simulink model "pressingswitch_fan"  (R2021a)
settings: Solver=FixedStepAuto  StartTime=0.0  StopTime=inf  FixedStep=0.01  RelTol=1e-3
libraries: simulink x1
settings Model: Creator=surya  LastModifiedBy=surya

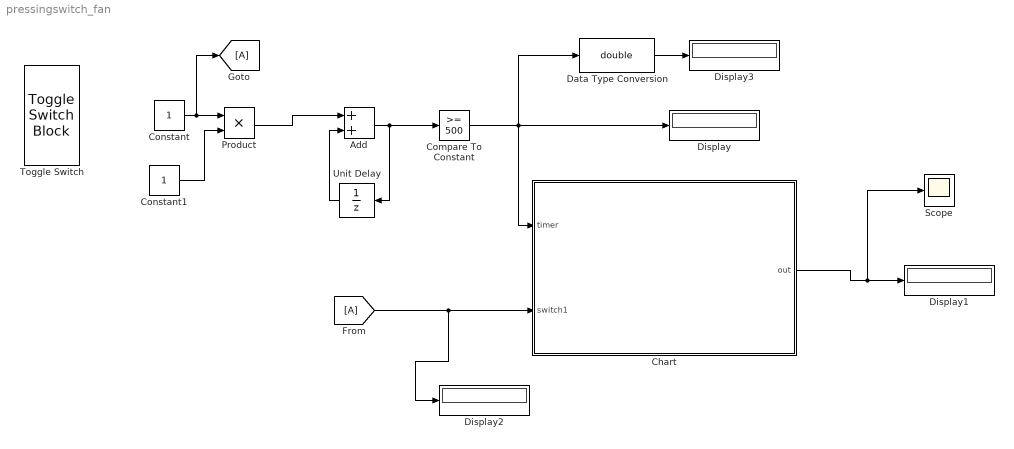
== system pressingswitch_fan ==
  Add : Sum
  Chart : Stateflow chart  TreatAsAtomicUnit=on
  Compare To Constant : simulink/Logic and Bit Operations/Compare To Constant  relop=>=  const=500  OutDataTypeStr=boolean
  Constant : Constant
  Constant1 : Constant
  Data Type Conversion : DataTypeConversion  OutDataTypeStr=double
  Display{,1..3} (4 alike) : Display
  Product : Product
  Scope : Scope
  Toggle Switch : ToggleSwitchBlock
      settings: Values={{'Off', 'On'}, [0 1]}
  Unit Delay : UnitDelay  SampleTime=-1  HasFrameUpgradeWarning=on
  wires:
  Unit Delay/1 -> Add/2
  Add/1 -> Unit Delay/1, Compare To Constant/1
  Constant/1 -> [A], Product/1
  Constant1/1 -> Product/2
  Product/1 -> Add/1
  Compare To Constant/1 -> Data Type Conversion/1, Display/1, Chart/1(timer)
  [A] -> Display2/1, Chart/2(switch1)
  Chart/1(out) -> Scope/1, Display1/1
  Data Type Conversion/1 -> Display3/1

== stateflow chart pressingswitch_fan/Chart ==
  state OFF
    en: out=0;
  state ON
    en:out=1;
  (default) -> OFF
  OFF -> ON : [timer==1 & switch1==1&after(1000,sec)]
  ON -> OFF : [timer==0 | switch1==0]
  data: timer input; switch1 input; out output
